simulink model "Temporal1_tmp"  (Simulink 8.3)
settings: Solver=ode45  StartTime=0.0  StopTime=20  RelTol=1e-3
settings Model: Creator=scaife  LastModifiedBy=bourbouh  CovSFcnEnable=on  ExtModeAutoUpdateStatusClock=off
settings DataIOCC: SignalLoggingName=sigsOut
settings DebuggingCC: SaveWithParameterizedLinksMsg=none  SignalResolutionControl=TryResolveAllWithWarning  SolverPrmCheckMsg=none  MultiTaskDSMMsg=warning  MultiTaskCondExecSysMsg=none  FrameProcessingCompatibilityMsg=error  StateNameClashWarn=none
settings HardwareCC: TargetUnknown=on
settings SFSimCC: SimParseCustomCode=off
settings GRTTargetCC: GeneratePreprocessorConditionals=Use local settings

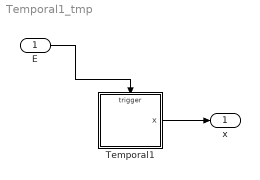
== system Temporal1_tmp ==
  E : Inport
  Temporal1 : Stateflow chart  TreatAsAtomicUnit=on
      settings: PermitHierarchicalResolution=ParametersOnly
  x : Outport
  wires:
  E/1 -> Temporal1/Trigger
  Temporal1/1(x) -> x/1

== stateflow chart Temporal1 ==
  state A/
    en : x++;
  state B/
    en : x++;
  (default) -> A
  A -> B : E[after(2,E)]
  B -> A : after(3,E)
  data: x output int32
  events: E input RISING_EDGE_EVENT
